simulink model "six_plus_six_AcmsteeringV09_main_2lfrf"  (R2014a)
settings: Solver=FixedStepDiscrete  StartTime=0.0  StopTime=10.0  FixedStep=0.0005  RelTol=1e-3
InitFcn:
  | Veh_Par_wxt
undefined symbols (not defined in the file or in its folder): acc_spdctl, ag_thr, B, bra_em, bra_pre_gz2, bra_pre_gz34, bra_pre_yd, brakepre_dem_data, brakeTrq_dem_data, bratrq_max, ecucoder_acal, eff_tran, ESP_switch, G, guzhang_lf, guzhang_lm, guzhang_lr, guzhang_rf, guzhang_rm, guzhang_rr, kd1, kd2, ki1, ki2, kp1, kp2, L, myFIS, premax, Radius, RC_switch, s_opt_yi, s_opt_zhuan, s_opt_zhuan_add, s_opt_zhuan_table, spd_map_mot, spd_spdctl, speed_thr_park, TCS_switch, tras_ratio, trq_map_mot, trqmax_yd, trqmax_zx, trqmaxneg, v_gain, v_table, v_thr_park, zhidong_bianmazhi, zhidong_down, zhidong_up, zhidong_youmen, zhuanxiang_bianmazhi, zhuanxiang_down, zhuanxiang_up, zhuanxiang_youmen
libraries: simulink x980, ec5744lib x59, fuzblock x2
(part 3 of 25)

== system six_plus_six_AcmsteeringV09_main_2lfrf/Data_input/MCU2_1 ==
  In1 : Inport
  In2 : Inport  Port=2
  Trigger : TriggerPort  TriggerType=function-call  PortDimensions=1
  MCU2 : Subsystem
  MCU2_MotorStallingFault : Outport
  MCU2_UdcDetectionFault : Outport  Port=2
  MCU2_TempSensorFault : Outport  Port=3
  MCU2_ActiveDischargingFault : Outport  Port=4
  MCU2_ldcSensorFault : Outport  Port=5
  MCU2_luSensorFault : Outport  Port=6
  MCU2_lvSensorFault : Outport  Port=7
  MCU2_FaultLevel : Outport  Port=8
  MCU2_Controllerload : Outport  Port=9
  MCU2_CanCommunicationFault : Outport  Port=10
  MCU2_MemoryFault : Outport  Port=11
  MCU2_DownratingFault : Outport  Port=12
  MCU2_IGBTFault : Outport  Port=13
  MCU2_MotorOverTemp : Outport  Port=14
  MCU2_ControllerOverTemp : Outport  Port=15
  MCU2_MotorOverSpeed : Outport  Port=16
  MCU2_RotaryInverterFault : Outport  Port=17
  MCU2_UnderVoltage : Outport  Port=18
  MCU2_OverVoltage : Outport  Port=19
  MCU2_MotorOverLoad : Outport  Port=20
  wires:
  MCU2/1(MCU2_MotorStallingFault_Out) -> MCU2_MotorStallingFault/1
  MCU2/7(MCU2_IvSensorFault_Out) -> MCU2_lvSensorFault/1
  MCU2/4(MCU2_ActieDischargingFault_Out) -> MCU2_ActiveDischargingFault/1
  MCU2/12(MCU2_DownratingFault_Out) -> MCU2_DownratingFault/1
  MCU2/13(MCU2_IGBTFault_Out) -> MCU2_IGBTFault/1
  MCU2/3(MCU2_TempSensorFault_Out) -> MCU2_TempSensorFault/1
  MCU2/10(MCU2_CanCommunicationFault_Out) -> MCU2_CanCommunicationFault/1
  MCU2/11(MCU2_MemoryFault_Out) -> MCU2_MemoryFault/1
  MCU2/14(MCU2_MotorOverTemp_Out) -> MCU2_MotorOverTemp/1
  MCU2/2(MCU2_UdcDetectionFault_Out) -> MCU2_UdcDetectionFault/1
  MCU2/5(MCU2_IdcSensorFault_Out) -> MCU2_ldcSensorFault/1
  In2/1 -> MCU2/1(input)
  In1/1 -> MCU2/Enable
  MCU2/6(MCU2_IuSensorFault_Out) -> MCU2_luSensorFault/1
  MCU2/8(MCU2_FaultLevel_Out) -> MCU2_FaultLevel/1
  MCU2/9(MCU2_ControllerOverload_Out) -> MCU2_Controllerload/1
  MCU2/20(MCU2_MotorOverLoad_Out) -> MCU2_MotorOverLoad/1
  MCU2/18(MCU2_UnderVoltage_Out) -> MCU2_UnderVoltage/1
  MCU2/19(MCU2_OverVoltage_Out) -> MCU2_OverVoltage/1
  MCU2/15(MCU2_ControllerOverTemp_Out) -> MCU2_ControllerOverTemp/1
  MCU2/16(MCU2_MotorOverSpeed_Out) -> MCU2_MotorOverSpeed/1
  MCU2/17(MCU2_RotaryInverterFault_Out) -> MCU2_RotaryInverterFault/1

== matlab function six_plus_six_AcmsteeringV09_main_2lfrf/MainControl/mode_control/backward/backward/Drive/驱动防滑控制TCS/直行TCS/直行/MATLAB Function7 ==
  data: trq_dem_lf input; trq_dem_lm input; trq_dem_lr input; trq_dem_rf input; trq_dem_rm input; trq_dem_rr input; bra_pre_l input; bra_pre_r input; brake_dem input; flag_lf input; flag_lm input; flag_lr input; trq_out_lf output; trq_out_lm output; flag_rf input; flag_rm input; flag_rr input; trq_out_lr output; trq_out_rf output; trq_out_rm output; trq_out_rr output; trq_pid_lf input; trq_pid_lm input; trq_pid_lr input; trq_pid_rf input; trq_pid_rm input; trq_pid_rr input; brapre_out_l output; brapre_out_r output; mode output
function [trq_out_lf,trq_out_lm,trq_out_lr,trq_out_rf,trq_out_rm,trq_out_rr,brapre_out_l,brapre_out_r,mode] = fcn(trq_dem_lf,trq_dem_lm,trq_dem_lr,trq_dem_rf,trq_dem_rm,trq_dem_rr,bra_pre_l,bra_pre_r,brake_dem,flag_lf,flag_lm,flag_lr,flag_rf,flag_rm,flag_rr,trq_pid_lf,trq_pid_lm,trq_pid_lr,trq_pid_rf,trq_pid_rm,trq_pid_rr)
%#codegen pid模块在外面做，里面进行十六种情况的判断，先看一下效果，不能再修改。
if flag_lf==0 && flag_lm==0 && flag_lr==0 && flag_rf==0 && flag_rm==0 && flag_rr==0 % 0电机滑转===============================================0电机滑转
    trq_out_lf=single(trq_dem_lf);
    trq_out_lm=single(trq_dem_lm);
    trq_out_lr=single(trq_dem_lr);
    trq_out_rf=single(trq_dem_rf);
    trq_out_rm=single(trq_dem_rm);
    trq_out_rr=single(trq_dem_rr);
    brapre_out_l=single(bra_pre_l+brake_dem);
    brapre_out_r=single(bra_pre_r+brake_dem);
    mode=int8(1);
    
    
    
    
    
    
    
    
    
elseif flag_lf==1 && flag_lm==0 && flag_lr==0 && flag_rf==0 && flag_rm==0 && flag_rr==0 %左前轮滑转===================================================1电机滑转
    trq_out_lf=single(trq_pid_lf);
    trq_out_lm=single(trq_dem_lm+(trq_dem_lf-trq_out_lf)/2);
    trq_out_lr=single(trq_dem_lr+(trq_dem_lf-trq_out_lf)/2);
    trq_out_rf=single(trq_dem_rf);
    trq_out_rm=single(trq_dem_rm);
    trq_out_rr=single(trq_dem_rr);
    brapre_out_l=single(bra_pre_l+brake_dem);
    brapre_out_r=single(bra_pre_r+brake_dem);
    mode=int8(2);
elseif flag_lf==0 && flag_lm==1 && flag_lr==0 && flag_rf==0 && flag_rm==0 && flag_rr==0 %左中轮滑转
    trq_out_lm=single(trq_pid_lm);
    trq_out_lf=single(trq_dem_lf+(trq_dem_lm-trq_out_lm)/2);
    trq_out_lr=single(trq_dem_lr+(trq_dem_lm-trq_out_lm)/2);
    trq_out_rf=single(trq_dem_rf);
    trq_out_rm=single(trq_dem_rm);
    trq_out_rr=single(trq_dem_rr);
    brapre_out_l=single(bra_pre_l+brake_dem);
    brapre_out_r=single(bra_pre_r+brake_dem);
    mode=int8(3);
elseif flag_lf==0 && flag_lm==0 && flag_lr==1 && flag_rf==0 && flag_rm==0 && flag_rr==0 %左后轮滑转
    trq_out_lr=single(trq_pid_lr);
    trq_out_lf=single(trq_dem_lf+(trq_dem_lr-trq_out_lr)/2);
    trq_out_lm=single(trq_dem_lm+(trq_dem_lr-trq_out_lr)/2);
    trq_out_rf=single(trq_dem_rf);
    trq_out_rm=single(trq_dem_rm);
    trq_out_rr=single(trq_dem_rr);
    brapre_out_l=single(bra_pre_l+brake_dem);
    brapre_out_r=single(bra_pre_r+brake_dem);
    mode=int8(4);
    
elseif flag_lf==0 && flag_lm==0 && flag_lr==0 && flag_rf==1 && flag_rm==0 && flag_rr==0 %右前轮滑转
    trq_out_rf=single(trq_pid_rf);
    trq_out_rm=single(trq_dem_rm+(trq_dem_rf-trq_out_rf)/2);
    trq_out_rr=single(trq_dem_rr+(trq_dem_rf-trq_out_rf)/2);
    trq_out_lf=single(trq_dem_lf);
    trq_out_lm=single(trq_dem_lm);
    trq_out_lr=single(trq_dem_lr);
    brapre_out_l=single(bra_pre_l+brake_dem);
    brapre_out_r=single(bra_pre_r+brake_dem);
    mode=int8(5);
elseif flag_lf==0 && flag_lm==0 && flag_lr==0 && flag_rf==0 && flag_rm==1 && flag_rr==0 %右中轮滑转
    trq_out_rm=single(trq_pid_rm);
    trq_out_rf=single(trq_dem_rf+(trq_dem_rm-trq_out_rm)/2);
    trq_out_rr=single(trq_dem_rr+(trq_dem_rm-trq_out_rm)/2);
    trq_out_lf=single(trq_dem_lf);
    trq_out_lm=single(trq_dem_lm);
    trq_out_lr=single(trq_dem_lr);
    brapre_out_l=single(bra_pre_l+brake_dem);
    brapre_out_r=single(bra_pre_r+brake_dem);
    mode=int8(6);
elseif flag_lf==0 && flag_lm==0 && flag_lr==0 && flag_rf==0 && flag_rm==0 && flag_rr==1 %右后轮滑转
    trq_out_rr=single(trq_pid_rr);
    trq_out_rf=single(trq_dem_rf+(trq_dem_rr-trq_out_rr)/2);
    trq_out_rm=single(trq_dem_rm+(trq_dem_rr-trq_out_rr)/2);
    trq_out_lf=single(trq_dem_lf);
    trq_out_lm=single(trq_dem_lm);
    trq_out_lr=single(trq_dem_lr);
    brapre_out_l=single(bra_pre_l+brake_dem);
    brapre_out_r=single(bra_pre_r+brake_dem);
    mode=int8(7);
    
    
    
    
    
    
    
    
    
    
elseif flag_lf==1 && flag_lm==1 && flag_lr==0 && flag_rf==0 && flag_rm==0 && flag_rr==0 %左前-左中 轮滑转===================================================2电机滑转    左侧
    trq_out_lf=single(trq_pid_lf);
    trq_out_lm=single(trq_pid_lm);
    trq_out_lr=single(trq_dem_lr+(trq_dem_lf-trq_out_lf)+(trq_dem_lm-trq_out_lm));
    trq_out_rf=single(trq_dem_rf);
    trq_out_rm=single(trq_dem_rm);
    trq_out_rr=single(trq_dem_rr);
    brapre_out_l=single(bra_pre_l+brake_dem);
    brapre_out_r=single(bra_pre_r+brake_dem);
    mode=int8(8);
elseif flag_lf==1 && flag_lm==0 && flag_lr==1 && flag_rf==0 && flag_rm==0 && flag_rr==0 %左前-左后 轮滑转
    trq_out_lf=single(trq_pid_lf);
    trq_out_lr=single(trq_pid_lr);
    trq_out_lm=single(trq_dem_lm+(trq_dem_lf-trq_out_lf)+(trq_dem_lr-trq_out_lr));
    trq_out_rf=single(trq_dem_rf);
    trq_out_rm=single(trq_dem_rm);
    trq_out_rr=single(trq_dem_rr);
    brapre_out_l=single(bra_pre_l+brake_dem);
    brapre_out_r=single(bra_pre_r+brake_dem);
    mode=int8(9);
elseif flag_lf==0 && flag_lm==1 && flag_lr==1 && flag_rf==0 && flag_rm==0 && flag_rr==0 %左中-左后 轮滑转
    trq_out_lm=single(trq_pid_lm);
    trq_out_lr=single(trq_pid_lr);
    trq_out_lf=single(trq_dem_lf+(trq_dem_lm-trq_out_lm)+(trq_dem_lr-trq_out_lr));
    trq_out_rf=single(trq_dem_rf);
    trq_out_rm=single(trq_dem_rm);
    trq_out_rr=single(trq_dem_rr);
    brapre_out_l=single(bra_pre_l+brake_dem);
    brapre_out_r=single(bra_pre_r+brake_dem);
    mode=int8(10);
    
elseif flag_lf==0 && flag_lm==0 && flag_lr==0 && flag_rf==1 && flag_rm==1 && flag_rr==0 %右前-右中 轮滑转                        右侧
    trq_out_rf=single(trq_pid_rf);
    trq_out_rm=single(trq_pid_rm);
    trq_out_rr=single(trq_dem_rr+(trq_dem_rf-trq_out_rf)+(trq_dem_rm-trq_out_rm));
    trq_out_lf=single(trq_dem_lf);
    trq_out_lm=single(trq_dem_lm);
    trq_out_lr=single(trq_dem_lr);
    brapre_out_l=single(bra_pre_l+brake_dem);
    brapre_out_r=single(bra_pre_r+brake_dem);
    mode=int8(11);
elseif flag_lf==0 && flag_lm==0 && flag_lr==0 && flag_rf==1 && flag_rm==0 && flag_rr==1 %右前-右后 轮滑转
    trq_out_rf=single(trq_pid_rf);
    trq_out_rr=single(trq_pid_rr);
    trq_out_rm=single(trq_dem_rm+(trq_dem_rf-trq_out_rf)+(trq_dem_rr-trq_out_rr));
    trq_out_lf=single(trq_dem_lf);
    trq_out_lm=single(trq_dem_lm);
    trq_out_lr=single(trq_dem_lr);
    brapre_out_l=single(bra_pre_l+brake_dem);
    brapre_out_r=single(bra_pre_r+brake_dem);
    mode=int8(12);
elseif flag_lf==0 && flag_lm==0 && flag_lr==0 && flag_rf==0 && flag_rm==1 && flag_rr==1 %右中-右后 轮滑转
    trq_out_rm=single(trq_pid_rm);
    trq_out_rr=single(trq_pid_rr);
    trq_out_rf=single(trq_dem_rf+(trq_dem_rm-trq_out_rm)+(trq_dem_rr-trq_out_rr));
    trq_out_lf=single(trq_dem_lf);
    trq_out_lm=single(trq_dem_lm);
    trq_out_lr=single(trq_dem_lr);
    brapre_out_l=single(bra_pre_l+brake_dem);
    brapre_out_r=single(bra_pre_r+brake_dem);
    mode=int8(13);
    
elseif flag_lf==1 && flag_lm==0 && flag_lr==0 && flag_rf==1 && flag_rm==0 && flag_rr==0 %左前-右前 轮滑转                 对侧
    trq_out_lf=single(trq_pid_lf);
    trq_out_lm=single(trq_dem_lm+(trq_dem_lf-trq_out_lf)/2);
    trq_out_lr=single(trq_dem_lr+(trq_dem_lf-trq_out_lf)/2);
    trq_out_rf=single(trq_pid_rf);
    trq_out_rm=single(trq_dem_rm+(trq_dem_rf-trq_out_rf)/2);
    trq_out_rr=single(trq_dem_rr+(trq_dem_rf-trq_out_rf)/2);
    brapre_out_l=single(bra_pre_l+brake_dem);
    brapre_out_r=single(bra_pre_r+brake_dem);
    mode=int8(14);
elseif flag_lf==1 && flag_lm==0 && flag_lr==0 && flag_rf==0 && flag_rm==1 && flag_rr==0 %左前-右中 轮滑转
    trq_out_lf=single(trq_pid_lf);
    trq_out_lm=single(trq_dem_lm+(trq_dem_lf-trq_out_lf)/2);
    trq_out_lr=single(trq_dem_lr+(trq_dem_lf-trq_out_lf)/2);
    trq_out_rm=single(trq_pid_rm);
    trq_out_rf=single(trq_dem_rf+(trq_dem_rm-trq_out_rm)/2);
    trq_out_rr=single(trq_dem_rr+(trq_dem_rm-trq_out_rm)/2);
    brapre_out_l=single(bra_pre_l+brake_dem);
    brapre_out_r=single(bra_pre_r+brake_dem);
    mode=int8(15);
elseif flag_lf==1 && flag_lm==0 && flag_lr==0 && flag_rf==0 && flag_rm==0 && flag_rr==1 %左前-右后 轮滑转
    trq_out_lf=single(trq_pid_lf);
    trq_out_lm=single(trq_dem_lm+(trq_dem_lf-trq_out_lf)/2);
    trq_out_lr=single(trq_dem_lr+(trq_dem_lf-trq_out_lf)/2);
    trq_out_rr=single(trq_pid_rr);
    trq_out_rf=single(trq_dem_rf+(trq_dem_rr-trq_out_rr)/2);
    trq_out_rm=single(trq_dem_rm+(trq_dem_rr-trq_out_rr)/2);
    brapre_out_l=single(bra_pre_l+brake_dem);
    brapre_out_r=single(bra_pre_r+brake_dem);
    mode=int8(16);
    
elseif flag_lf==0 && flag_lm==1 && flag_lr==0 && flag_rf==1 && flag_rm==0 && flag_rr==0 %左中-右前 轮滑转                 对侧
    trq_out_lm=single(trq_pid_lm);
    trq_out_lf=single(trq_dem_lf+(trq_dem_lm-trq_out_lm)/2);
    trq_out_lr=single(trq_dem_lr+(trq_dem_lm-trq_out_lm)/2);
    trq_out_rf=single(trq_pid_rf);
    trq_out_rm=single(trq_dem_rm+(trq_dem_rf-trq_out_rf)/2);
    trq_out_rr=single(trq_dem_rr+(trq_dem_rf-trq_out_rf)/2);
    brapre_out_l=single(bra_pre_l+brake_dem);
    brapre_out_r=single(bra_pre_r+brake_dem);
    mode=int8(17);
elseif flag_lf==0 && flag_lm==1 && flag_lr==0 && flag_rf==0 && flag_rm==1 && flag_rr==0 %左中-右中 轮滑转
    trq_out_lm=single(trq_pid_lm);
    trq_out_lf=single(trq_dem_lf+(trq_dem_lm-trq_out_lm)/2);
    trq_out_lr=single(trq_dem_lr+(trq_dem_lm-trq_out_lm)/2);
    trq_out_rm=single(trq_pid_rm);
    trq_out_rf=single(trq_dem_rf+(trq_dem_rm-trq_out_rm)/2);
    trq_out_rr=single(trq_dem_rr+(trq_dem_rm-trq_out_rm)/2);
    brapre_out_l=single(bra_pre_l+brake_dem);
    brapre_out_r=single(bra_pre_r+brake_dem);
    mode=int8(18);
elseif flag_lf==0 && flag_lm==1 && flag_lr==0 && flag_rf==0 && flag_rm==0 && flag_rr==1 %左中-右后 轮滑转
    trq_out_lm=single(trq_pid_lm);
    trq_out_lf=single(trq_dem_lf+(trq_dem_lm-trq_out_lm)/2);
    trq_out_lr=single(trq_dem_lr+(trq_dem_lm-trq_out_lm)/2);
    trq_out_rr=single(trq_pid_rr);
    trq_out_rf=single(trq_dem_rf+(trq_dem_rr-trq_out_rr)/2);
    trq_out_rm=single(trq_dem_rm+(trq_dem_rr-trq_out_rr)/2);
    brapre_out_l=single(bra_pre_l+brake_dem);
    brapre_out_r=single(bra_pre_r+brake_dem);
    mode=int8(19);
elseif flag_lf==0 && flag_lm==0 && flag_lr==1 && flag_rf==1 && flag_rm==0 && flag_rr==0 %左后-右前 轮滑转                 对侧
    trq_out_lr=single(trq_pid_lr);
    trq_out_lf=single(trq_dem_lf+(trq_dem_lr-trq_out_lr)/2);
    trq_out_lm=single(trq_dem_lm+(trq_dem_lr-trq_out_lr)/2);
    trq_out_rf=single(trq_pid_rf);
    trq_out_rm=single(trq_dem_rm+(trq_dem_rf-trq_out_rf)/2);
    trq_out_rr=single(trq_dem_rr+(trq_dem_rf-trq_out_rf)/2);
    brapre_out_l=single(bra_pre_l+brake_dem);
    brapre_out_r=single(bra_pre_r+brake_dem);
    mode=int8(20);
elseif flag_lf==0 && flag_lm==0 && flag_lr==1 && flag_rf==0 && flag_rm==1 && flag_rr==0 %左后-右中 轮滑转
    trq_out_lr=single(trq_pid_lr);
    trq_out_lf=single(trq_dem_lf+(trq_dem_lr-trq_out_lr)/2);
    trq_out_lm=single(trq_dem_lm+(trq_dem_lr-trq_out_lr)/2);
    trq_out_rm=single(trq_pid_rm);
    trq_out_rf=single(trq_dem_rf+(trq_dem_rm-trq_out_rm)/2);
    trq_out_rr=single(trq_dem_rr+(trq_dem_rm-trq_out_rm)/2);
    brapre_out_l=single(bra_pre_l+brake_dem);
    brapre_out_r=single(bra_pre_r+brake_dem);
    mode=int8(21);
elseif flag_lf==0 && flag_lm==0 && flag_lr==1 && flag_rf==0 && flag_rm==0 && flag_rr==1 %左后-右后 轮滑转
    trq_out_lr=single(trq_pid_lr);
    trq_out_lf=single(trq_dem_lf+(trq_dem_lr-trq_out_lr)/2);
    trq_out_lm=single(trq_dem_lm+(trq_dem_lr-trq_out_lr)/2);
    trq_out_rr=single(trq_pid_rr);
    trq_out_rf=single(trq_dem_rf+(trq_dem_rr-trq_out_rr)/2);
    trq_out_rm=single(trq_dem_rm+(trq_dem_rr-trq_out_rr)/2);
    brapre_out_l=single(bra_pre_l+brake_dem);
    brapre_out_r=single(bra_pre_r+brake_dem);
    mode=int8(22);
    
    
    
    
    
    
    
    
    
    
    
    
    
    
    
    
    
    
    
    
    
    
elseif flag_lf==1 && flag_lm==1 && flag_lr==1 && flag_rf==0 && flag_rm==0 && flag_rr==0 %左前-左中-左后 轮滑转===================================================3电机滑转    左侧
    trq_out_lf=single(trq_pid_lf);
    trq_out_lm=single(trq_pid_lm);
    trq_out_lr=single(trq_pid_lr);
    trq_out_rf=single(trq_dem_rf-((trq_dem_lf-trq_out_lf)+(trq_dem_lm-trq_out_lm)+(trq_dem_lr-trq_out_lr))/3);
    trq_out_rm=single(trq_dem_rm-((trq_dem_lf-trq_out_lf)+(trq_dem_lm-trq_out_lm)+(trq_dem_lr-trq_out_lr))/3);
    trq_out_rr=single(trq_dem_rr-((trq_dem_lf-trq_out_lf)+(trq_dem_lm-trq_out_lm)+(trq_dem_lr-trq_out_lr))/3);
    brapre_out_l=single(bra_pre_l+brake_dem);
    brapre_out_r=single(bra_pre_r+brake_dem);
    mode=int8(23);
elseif flag_lf==0 && flag_lm==0 && flag_lr==0 && flag_rf==1 && flag_rm==1 && flag_rr==1 %右前-右中-右后 轮滑转                      右侧
    trq_out_rf=single(trq_pid_rf);
    trq_out_rm=single(trq_pid_rm);
    trq_out_rr=single(trq_pid_rr);
    trq_out_lf=single(trq_dem_lf-((trq_dem_rf-trq_out_rf)+(trq_dem_rm-trq_out_rm)+(trq_dem_rr-trq_out_rr))/3);
    trq_out_lm=single(trq_dem_lm-((trq_dem_rf-trq_out_rf)+(trq_dem_rm-trq_out_rm)+(trq_dem_rr-trq_out_rr))/3);
    trq_out_lr=single(trq_dem_lr-((trq_dem_rf-trq_out_rf)+(trq_dem_rm-trq_out_rm)+(trq_dem_rr-trq_out_rr))/3);
    brapre_out_l=single(bra_pre_l+brake_dem);
    brapre_out_r=single(bra_pre_r+brake_dem);
    mode=int8(24);
    
elseif flag_lf==1 && flag_lm==1 && flag_lr==0 && flag_rf==1 && flag_rm==0 && flag_rr==0 %左前-左中-右前 轮滑转
    trq_out_lf=single(trq_pid_lf);
    trq_out_lm=single(trq_pid_lm);
    trq_out_lr=single(trq_dem_lr+(trq_dem_lf-trq_out_lf)+(trq_dem_lm-trq_out_lm));
    trq_out_rf=single(trq_pid_rf);
    trq_out_rm=single(trq_dem_rm+(trq_dem_rf-trq_out_rf)/2);
    trq_out_rr=single(trq_dem_rr+(trq_dem_rf-trq_out_rf)/2);
    brapre_out_l=single(bra_pre_l+brake_dem);
    brapre_out_r=single(bra_pre_r+brake_dem);
    mode=int8(25);
elseif flag_lf==1 && flag_lm==1 && flag_lr==0 && flag_rf==0 && flag_rm==1 && flag_rr==0 %左前-左中-右中 轮滑转
    trq_out_lf=single(trq_pid_lf);
    trq_out_lm=single(trq_pid_lm);
    trq_out_lr=single(trq_dem_lr+(trq_dem_lf-trq_out_lf)+(trq_dem_lm-trq_out_lm));
    trq_out_rm=single(trq_pid_rm);
    trq_out_rf=single(trq_dem_rf+(trq_dem_rm-trq_out_rm)/2);
    trq_out_rr=single(trq_dem_rr+(trq_dem_rm-trq_out_rm)/2);
    brapre_out_l=single(bra_pre_l+brake_dem);
    brapre_out_r=single(bra_pre_r+brake_dem);
    mode=int8(26);
elseif flag_lf==1 && flag_lm==1 && flag_lr==0 && flag_rf==0 && flag_rm==0 && flag_rr==1 %左前-左中-右后 轮滑转
    trq_out_lf=single(trq_pid_lf);
    trq_out_lm=single(trq_pid_lm);
    trq_out_lr=single(trq_dem_lr+(trq_dem_lf-trq_out_lf)+(trq_dem_lm-trq_out_lm));
    trq_out_rr=single(trq_pid_rr);
    trq_out_rf=single(trq_dem_rf+(trq_dem_rr-trq_out_rr)/2);
    trq_out_rm=single(trq_dem_rm+(trq_dem_rr-trq_out_rr)/2);
    brapre_out_l=single(bra_pre_l+brake_dem);
    brapre_out_r=single(bra_pre_r+brake_dem);
    mode=int8(27);
    
elseif flag_lf==1 && flag_lm==0 && flag_lr==1 && flag_rf==1 && flag_rm==0 && flag_rr==0 %左前-左后-右前 轮滑转
    trq_out_lf=single(trq_pid_lf);
    trq_out_lr=single(trq_pid_lr);
    trq_out_lm=single(trq_dem_lm+(trq_dem_lf-trq_out_lf)+(trq_dem_lr-trq_out_lr));
    trq_out_rf=single(trq_pid_rf);
    trq_out_rm=single(trq_dem_rm+(trq_dem_rf-trq_out_rf)/2);
    trq_out_rr=single(trq_dem_rr+(trq_dem_rf-trq_out_rf)/2);
    brapre_out_l=single(bra_pre_l+brake_dem);
    brapre_out_r=single(bra_pre_r+brake_dem);
    mode=int8(28);
elseif flag_lf==1 && flag_lm==0 && flag_lr==1 && flag_rf==0 && flag_rm==1 && flag_rr==0 %左前-左后-右中 轮滑转
    trq_out_lf=single(trq_pid_lf);
    trq_out_lr=single(trq_pid_lr);
    trq_out_lm=single(trq_dem_lm+(trq_dem_lf-trq_out_lf)+(trq_dem_lr-trq_out_lr));
    trq_out_rm=single(trq_pid_rm);
    trq_out_rf=single(trq_dem_rf+(trq_dem_rm-trq_out_rm)/2);
    trq_out_rr=single(trq_dem_rr+(trq_dem_rm-trq_out_rm)/2);
    brapre_out_l=single(bra_pre_l+brake_dem);
    brapre_out_r=single(bra_pre_r+brake_dem);
    mode=int8(29);
elseif flag_lf==1 && flag_lm==0 && flag_lr==1 && flag_rf==0 && flag_rm==0 && flag_rr==1 %左前-左后-右后 轮滑转
    trq_out_lf=single(trq_pid_lf);
    trq_out_lr=single(trq_pid_lr);
    trq_out_lm=single(trq_dem_lm+(trq_dem_lf-trq_out_lf)+(trq_dem_lr-trq_out_lr));
    trq_out_rr=single(trq_pid_rr);
    trq_out_rf=single(trq_dem_rf+(trq_dem_rr-trq_out_rr)/2);
    trq_out_rm=single(trq_dem_rm+(trq_dem_rr-trq_out_rr)/2);
    brapre_out_l=single(bra_pre_l+brake_dem);
    brapre_out_r=single(bra_pre_r+brake_dem);
    mode=int8(30);
    
elseif flag_lf==0 && flag_lm==1 && flag_lr==1 && flag_rf==1 && flag_rm==0 && flag_rr==0 %左中-左后-右前 轮滑转
    trq_out_lm=single(trq_pid_lm);
    trq_out_lr=single(trq_pid_lr);
    trq_out_lf=single(trq_dem_lf+(trq_dem_lm-trq_out_lm)+(trq_dem_lr-trq_out_lr));
    trq_out_rf=single(trq_pid_rf);
    trq_out_rm=single(trq_dem_rm+(trq_dem_rf-trq_out_rf)/2);
    trq_out_rr=single(trq_dem_rr+(trq_dem_rf-trq_out_rf)/2);
    brapre_out_l=single(bra_pre_l+brake_dem);
    brapre_out_r=single(bra_pre_r+brake_dem);
    mode=int8(31);
elseif flag_lf==0 && flag_lm==1 && flag_lr==1 && flag_rf==0 && flag_rm==1 && flag_rr==0 %左中-左后-右中 轮滑转
    trq_out_lm=single(trq_pid_lm);
    trq_out_lr=single(trq_pid_lr);
    trq_out_lf=single(trq_dem_lf+(trq_dem_lm-trq_out_lm)+(trq_dem_lr-trq_out_lr));
    trq_out_rm=single(trq_pid_rm);
    trq_out_rf=single(trq_dem_rf+(trq_dem_rm-trq_out_rm)/2);
    trq_out_rr=single(trq_dem_rr+(trq_dem_rm-trq_out_rm)/2);
    brapre_out_l=single(bra_pre_l+brake_dem);
    brapre_out_r=single(bra_pre_r+brake_dem);
    mode=int8(32);
elseif flag_lf==0 && flag_lm==1 && flag_lr==1 && flag_rf==0 && flag_rm==0 && flag_rr==1 %左中-左后-右后 轮滑转
    trq_out_lm=single(trq_pid_lm);
    trq_out_lr=single(trq_pid_lr);
    trq_out_lf=single(trq_dem_lf+(trq_dem_lm-trq_out_lm)+(trq_dem_lr-trq_out_lr));
    trq_out_rr=single(trq_pid_rr);
    trq_out_rf=single(trq_dem_rf+(trq_dem_rr-trq_out_rr)/2);
    trq_out_rm=single(trq_dem_rm+(trq_dem_rr-trq_out_rr)/2);
    brapre_out_l=single(bra_pre_l+brake_dem);
    brapre_out_r=single(bra_pre_r+brake_dem);
    mode=int8(33);
    
elseif flag_lf==1 && flag_lm==0 && flag_lr==0 && flag_rf==1 && flag_rm==1 && flag_rr==0 %右前-右中-左前 轮滑转
    trq_out_rf=single(trq_pid_rf);
    trq_out_rm=single(trq_pid_rm);
    trq_out_rr=single(trq_dem_rr+(trq_dem_rf-trq_out_rf)+(trq_dem_rm-trq_out_rm));
    trq_out_lf=single(trq_pid_lf);
    trq_out_lm=single(trq_dem_lm+(trq_dem_lf-trq_out_lf)/2);
    trq_out_lr=single(trq_dem_lr+(trq_dem_lf-trq_out_lf)/2);
    brapre_out_l=single(bra_pre_l+brake_dem);
    brapre_out_r=single(bra_pre_r+brake_dem);
    mode=int8(34);
elseif flag_lf==0 && flag_lm==1 && flag_lr==0 && flag_rf==1 && flag_rm==1 && flag_rr==0 %右前-右中-左中 轮滑转
    trq_out_rf=single(trq_pid_rf);
    trq_out_rm=single(trq_pid_rm);
    trq_out_rr=single(trq_dem_rr+(trq_dem_rf-trq_out_rf)+(trq_dem_rm-trq_out_rm));
    trq_out_lm=single(trq_pid_lm);
    trq_out_lf=single(trq_dem_lf+(trq_dem_lm-trq_out_lm)/2);
    trq_out_lr=single(trq_dem_lr+(trq_dem_lm-trq_out_lm)/2);
    brapre_out_l=single(bra_pre_l+brake_dem);
    brapre_out_r=single(bra_pre_r+brake_dem);
    mode=int8(35);
elseif flag_lf==0 && flag_lm==0 && flag_lr==1 && flag_rf==1 && flag_rm==1 && flag_rr==0 %右前-右中-左后 轮滑转
    trq_out_rf=single(trq_pid_rf);
    trq_out_rm=single(trq_pid_rm);
    trq_out_rr=single(trq_dem_rr+(trq_dem_rf-trq_out_rf)+(trq_dem_rm-trq_out_rm));
    trq_out_lr=single(trq_pid_lr);
    trq_out_lf=single(trq_dem_lf+(trq_dem_lr-trq_out_lr)/2);
    trq_out_lm=single(trq_dem_lm+(trq_dem_lr-trq_out_lr)/2);
    brapre_out_l=single(bra_pre_l+brake_dem);
    brapre_out_r=single(bra_pre_r+brake_dem);
    mode=int8(36);
    
elseif flag_lf==1 && flag_lm==0 && flag_lr==0 && flag_rf==1 && flag_rm==0 && flag_rr==1 %右前-右后-左前 轮滑转
    trq_out_rf=single(trq_pid_rf);
    trq_out_rr=single(trq_pid_rr);
    trq_out_rm=single(trq_dem_rm+(trq_dem_rf-trq_out_rf)+(trq_dem_rr-trq_out_rr));
    trq_out_lf=single(trq_pid_lf);
    trq_out_lm=single(trq_dem_lm+(trq_dem_lf-trq_out_lf)/2);
    trq_out_lr=single(trq_dem_lr+(trq_dem_lf-trq_out_lf)/2);
    brapre_out_l=single(bra_pre_l+brake_dem);
    brapre_out_r=single(bra_pre_r+brake_dem);
    mode=int8(37);
elseif flag_lf==0 && flag_lm==1 && flag_lr==0 && flag_rf==1 && flag_rm==0 && flag_rr==1 %右前-右后-左中 轮滑转
    trq_out_rf=single(trq_pid_rf);
    trq_out_rr=single(trq_pid_rr);
    trq_out_rm=single(trq_dem_rm+(trq_dem_rf-trq_out_rf)+(trq_dem_rr-trq_out_rr));
    trq_out_lm=single(trq_pid_lm);
    trq_out_lf=single(trq_dem_lf+(trq_dem_lm-trq_out_lm)/2);
    trq_out_lr=single(trq_dem_lr+(trq_dem_lm-trq_out_lm)/2);
    brapre_out_l=single(bra_pre_l+brake_dem);
    brapre_out_r=single(bra_pre_r+brake_dem);
    mode=int8(38);
elseif flag_lf==0 && flag_lm==0 && flag_lr==1 && flag_rf==1 && flag_rm==0 && flag_rr==1 %右前-右后-左后 轮滑转
    trq_out_rf=single(trq_pid_rf);
    trq_out_rr=single(trq_pid_rr);
    trq_out_rm=single(trq_dem_rm+(trq_dem_rf-trq_out_rf)+(trq_dem_rr-trq_out_rr));
    trq_out_lr=single(trq_pid_lr);
    trq_out_lf=single(trq_dem_lf+(trq_dem_lr-trq_out_lr)/2);
    trq_out_lm=single(trq_dem_lm+(trq_dem_lr-trq_out_lr)/2);
    brapre_out_l=single(bra_pre_l+brake_dem);
    brapre_out_r=single(bra_pre_r+brake_dem);
    mode=int8(39);
    
elseif flag_lf==1 && flag_lm==0 && flag_lr==0 && flag_rf==0 && flag_rm==1 && flag_rr==1 %右中-右后-左前 轮滑转
    trq_out_rm=single(trq_pid_rm);
    trq_out_rr=single(trq_pid_rr);
    trq_out_rf=single(trq_dem_rf+(trq_dem_rm-trq_out_rm)+(trq_dem_rr-trq_out_rr));
    trq_out_lf=single(trq_pid_lf);
    trq_out_lm=single(trq_dem_lm+(trq_dem_lf-trq_out_lf)/2);
    trq_out_lr=single(trq_dem_lr+(trq_dem_lf-trq_out_lf)/2);
    brapre_out_l=single(bra_pre_l+brake_dem);
    brapre_out_r=single(bra_pre_r+brake_dem);
    mode=int8(40);
elseif flag_lf==0 && flag_lm==1 && flag_lr==0 && flag_rf==0 && flag_rm==1 && flag_rr==1 %右中-右后-左中 轮滑转
    trq_out_rm=single(trq_pid_rm);
    trq_out_rr=single(trq_pid_rr);
    trq_out_rf=single(trq_dem_rf+(trq_dem_rm-trq_out_rm)+(trq_dem_rr-trq_out_rr));
    trq_out_lm=single(trq_pid_lm);
    trq_out_lf=single(trq_dem_lf+(trq_dem_lm-trq_out_lm)/2);
    trq_out_lr=single(trq_dem_lr+(trq_dem_lm-trq_out_lm)/2);
    brapre_out_l=single(bra_pre_l+brake_dem);
    brapre_out_r=single(bra_pre_r+brake_dem);
    mode=int8(41);
elseif flag_lf==0 && flag_lm==0 && flag_lr==1 && flag_rf==0 && flag_rm==1 && flag_rr==1 %右中-右后-左后 轮滑转
    trq_out_rm=single(trq_pid_rm);
    trq_out_rr=single(trq_pid_rr);
    trq_out_rf=single(trq_dem_rf+(trq_dem_rm-trq_out_rm)+(trq_dem_rr-trq_out_rr));
    trq_out_lr=single(trq_pid_lr);
    trq_out_lf=single(trq_dem_lf+(trq_dem_lr-trq_out_lr)/2);
    trq_out_lm=single(trq_dem_lm+(trq_dem_lr-trq_out_lr)/2);
    brapre_out_l=single(bra_pre_l+brake_dem);
    brapre_out_r=single(bra_pre_r+brake_dem);
    mode=int8(42);
    
    
    
    
    
    
    
    
    
    
    
    
    
    
    
    
    
    
    
    
    
elseif flag_lf==1 && flag_lm==1 && flag_lr==1 && flag_rf==1 && flag_rm==0 && flag_rr==0 %左前-左中-左后 右前 轮滑转===================================================4电机滑转
    trq_out_lf=single(trq_pid_lf);
    trq_out_lm=single(trq_pid_lm);
    trq_out_lr=single(trq_pid_lr);
    trq_out_rf=single(trq_pid_rf);
    trq_out_rm=single(trq_dem_rm-((trq_dem_lf-trq_out_lf)+(trq_dem_lm-trq_out_lm)+(trq_dem_lr-trq_out_lr)-(trq_dem_rf-trq_out_rf))/2);
    trq_out_rr=single(trq_dem_rr-((trq_dem_lf-trq_out_lf)+(trq_dem_lm-trq_out_lm)+(trq_dem_lr-trq_out_lr)-(trq_dem_rf-trq_out_rf))/2);
    brapre_out_l=single(bra_pre_l+brake_dem);
    brapre_out_r=single(bra_pre_r+brake_dem);
    mode=int8(43);
elseif flag_lf==1 && flag_lm==1 && flag_lr==1 && flag_rf==0 && flag_rm==1 && flag_rr==0 %左前-左中-左后 右中 轮滑转
    trq_out_lf=single(trq_pid_lf);
    trq_out_lm=single(trq_pid_lm);
    trq_out_lr=single(trq_pid_lr);
    trq_out_rm=single(trq_pid_rm);
    trq_out_rf=single(trq_dem_rf-((trq_dem_lf-trq_out_lf)+(trq_dem_lm-trq_out_lm)+(trq_dem_lr-trq_out_lr)-(trq_dem_rm-trq_out_rm))/2);
    trq_out_rr=single(trq_dem_rr-((trq_dem_lf-trq_out_lf)+(trq_dem_lm-trq_out_lm)+(trq_dem_lr-trq_out_lr)-(trq_dem_rm-trq_out_rm))/2);
    brapre_out_l=single(bra_pre_l+brake_dem);
    brapre_out_r=single(bra_pre_r+brake_dem);
    mode=int8(44);
elseif flag_lf==1 && flag_lm==1 && flag_lr==1 && flag_rf==0 && flag_rm==0 && flag_rr==1 %左前-左中-左后 右后 轮滑转
    trq_out_lf=single(trq_pid_lf);
    trq_out_lm=single(trq_pid_lm);
    trq_out_lr=single(trq_pid_lr);
    trq_out_rr=single(trq_pid_rr);
    trq_out_rf=single(trq_dem_rf-((trq_dem_lf-trq_out_lf)+(trq_dem_lm-trq_out_lm)+(trq_dem_lr-trq_out_lr)-(trq_dem_rr-trq_out_rr))/2);
    trq_out_rm=single(trq_dem_rm-((trq_dem_lf-trq_out_lf)+(trq_dem_lm-trq_out_lm)+(trq_dem_lr-trq_out_lr)-(trq_dem_rr-trq_out_rr))/2);
    brapre_out_l=single(bra_pre_l+brake_dem);
    brapre_out_r=single(bra_pre_r+brake_dem);
    mode=int8(45);
    
elseif flag_lf==1 && flag_lm==0 && flag_lr==0 && flag_rf==1 && flag_rm==1 && flag_rr==1 %右前-右中-右后 左前 轮滑转
    trq_out_rf=single(trq_pid_rf);
    trq_out_rm=single(trq_pid_rm);
    trq_out_rr=single(trq_pid_rr);
    trq_out_lf=single(trq_pid_lf);
    trq_out_lm=single(trq_dem_lm-((trq_dem_rf-trq_out_rf)+(trq_dem_rm-trq_out_rm)+(trq_dem_rr-trq_out_rr)-(trq_dem_lf-trq_out_lf))/2);
    trq_out_lr=single(trq_dem_lr-((trq_dem_rf-trq_out_rf)+(trq_dem_rm-trq_out_rm)+(trq_dem_rr-trq_out_rr)-(trq_dem_lf-trq_out_lf))/2);
    brapre_out_l=single(bra_pre_l+brake_dem);
    brapre_out_r=single(bra_pre_r+brake_dem);
    mode=int8(46);
elseif flag_lf==0 && flag_lm==1 && flag_lr==0 && flag_rf==1 && flag_rm==1 && flag_rr==1 %右前-右中-右后 左中 轮滑转
    trq_out_rf=single(trq_pid_rf);
    trq_out_rm=single(trq_pid_rm);
    trq_out_rr=single(trq_pid_rr);
    trq_out_lm=single(trq_pid_lm);
    trq_out_lf=single(trq_dem_lf-((trq_dem_rf-trq_out_rf)+(trq_dem_rm-trq_out_rm)+(trq_dem_rr-trq_out_rr)-(trq_dem_lm-trq_out_lm))/2);
    trq_out_lr=single(trq_dem_lr-((trq_dem_rf-trq_out_rf)+(trq_dem_rm-trq_out_rm)+(trq_dem_rr-trq_out_rr)-(trq_dem_lm-trq_out_lm))/2);
    brapre_out_l=single(bra_pre_l+brake_dem);
    brapre_out_r=single(bra_pre_r+brake_dem);
    mode=int8(47);
elseif flag_lf==0 && flag_lm==0 && flag_lr==1 && flag_rf==1 && flag_rm==1 && flag_rr==1 %右前-右中-右后 左后 轮滑转
    trq_out_rf=single(trq_pid_rf);
    trq_out_rm=single(trq_pid_rm);
    trq_out_rr=single(trq_pid_rr);
    trq_out_lr=single(trq_pid_lr);
    trq_out_lf=single(trq_dem_lf-((trq_dem_rf-trq_out_rf)+(trq_dem_rm-trq_out_rm)+(trq_dem_rr-trq_out_rr)-(trq_dem_lr-trq_out_lr))/2);
    trq_out_lm=single(trq_dem_lm-((trq_dem_rf-trq_out_rf)+(trq_dem_rm-trq_out_rm)+(trq_dem_rr-trq_out_rr)-(trq_dem_lr-trq_out_lr))/2);
    brapre_out_l=single(bra_pre_l+brake_dem);
    brapre_out_r=single(bra_pre_r+brake_dem);
    mode=int8(48);
    
elseif flag_lf==1 && flag_lm==1 && flag_lr==0 && flag_rf==1 && flag_rm==1 && flag_rr==0 %左前-左中 右前-右中 轮滑转
    trq_out_lf=single(trq_pid_lf);
    trq_out_lm=single(trq_pid_lm);
    trq_out_lr=single(trq_dem_lr+(trq_dem_lf-trq_out_lf)+(trq_dem_lm-trq_out_lm));
    trq_out_rf=single(trq_pid_rf);
    trq_out_rm=single(trq_pid_rm);
    trq_out_rr=single(trq_dem_rr+(trq_dem_rf-trq_out_rf)+(trq_dem_rm-trq_out_rm));
    brapre_out_l=single(bra_pre_l+brake_dem);
    brapre_out_r=single(bra_pre_r+brake_dem);
    mode=int8(49);
elseif flag_lf==1 && flag_lm==1 && flag_lr==0 && flag_rf==1 && flag_rm==0 && flag_rr==1 %左前-左中 右前-右后 轮滑转
    trq_out_lf=single(trq_pid_lf);
    trq_out_lm=single(trq_pid_lm);
    trq_out_lr=single(trq_dem_lr+(trq_dem_lf-trq_out_lf)+(trq_dem_lm-trq_out_lm));
    trq_out_rf=single(trq_pid_rf);
    trq_out_rr=single(trq_pid_rr);
    trq_out_rm=single(trq_dem_rm+(trq_dem_rf-trq_out_rf)+(trq_dem_rr-trq_out_rr));
    brapre_out_l=single(bra_pre_l+brake_dem);
    brapre_out_r=single(bra_pre_r+brake_dem);
    mode=int8(50);
elseif flag_lf==1 && flag_lm==1 && flag_lr==0 && flag_rf==0 && flag_rm==1 && flag_rr==1 %左前-左中 右中-右后 轮滑转
    trq_out_lf=single(trq_pid_lf);
    trq_out_lm=single(trq_pid_lm);
    trq_out_lr=single(trq_dem_lr+(trq_dem_lf-trq_out_lf)+(trq_dem_lm-trq_out_lm));
    trq_out_rm=single(trq_pid_rm);
    trq_out_rr=single(trq_pid_rr);
    trq_out_rf=single(trq_dem_rf+(trq_dem_rm-trq_out_rm)+(trq_dem_rr-trq_out_rr));
    brapre_out_l=single(bra_pre_l+brake_dem);
    brapre_out_r=single(bra_pre_r+brake_dem);
    mode=int8(51);
    
elseif flag_lf==1 && flag_lm==0 && flag_lr==1 && flag_rf==1 && flag_rm==1 && flag_rr==0 %左前-左后 右前-右中 轮滑转
    trq_out_lf=single(trq_pid_lf);
    trq_out_lr=single(trq_pid_lr);
    trq_out_lm=single(trq_dem_lm+(trq_dem_lf-trq_out_lf)+(trq_dem_lr-trq_out_lr));
    trq_out_rf=single(trq_pid_rf);
    trq_out_rm=single(trq_pid_rm);
    trq_out_rr=single(trq_dem_rr+(trq_dem_rf-trq_out_rf)+(trq_dem_rm-trq_out_rm));
    brapre_out_l=single(bra_pre_l+brake_dem);
    brapre_out_r=single(bra_pre_r+brake_dem);
    mode=int8(52);
elseif flag_lf==1 && flag_lm==0 && flag_lr==1 && flag_rf==1 && flag_rm==0 && flag_rr==1 %左前-左后 右前-右后 轮滑转
    trq_out_lf=single(trq_pid_lf);
    trq_out_lr=single(trq_pid_lr);
    trq_out_lm=single(trq_dem_lm+(trq_dem_lf-trq_out_lf)+(trq_dem_lr-trq_out_lr));
    trq_out_rf=single(trq_pid_rf);
    trq_out_rr=single(trq_pid_rr);
    trq_out_rm=single(trq_dem_rm+(trq_dem_rf-trq_out_rf)+(trq_dem_rr-trq_out_rr));
    brapre_out_l=single(bra_pre_l+brake_dem);
    brapre_out_r=single(bra_pre_r+brake_dem);
    mode=int8(53);
elseif flag_lf==1 && flag_lm==0 && flag_lr==1 && flag_rf==0 && flag_rm==1 && flag_rr==1 %左前-左后 右中-右后 轮滑转
    trq_out_lf=single(trq_pid_lf);
    trq_out_lr=single(trq_pid_lr);
    trq_out_lm=single(trq_dem_lm+(trq_dem_lf-trq_out_lf)+(trq_dem_lr-trq_out_lr));
    trq_out_rm=single(trq_pid_rm);
    trq_out_rr=single(trq_pid_rr);
    trq_out_rf=single(trq_dem_rf+(trq_dem_rm-trq_out_rm)+(trq_dem_rr-trq_out_rr));
    brapre_out_l=single(bra_pre_l+brake_dem);
    brapre_out_r=single(bra_pre_r+brake_dem);
    mode=int8(54);
    
elseif flag_lf==0 && flag_lm==1 && flag_lr==1 && flag_rf==1 && flag_rm==1 && flag_rr==0 %左中-左后 右前-右中 轮滑转
    trq_out_lm=single(trq_pid_lm);
    trq_out_lr=single(trq_pid_lr);
    trq_out_lf=single(trq_dem_lf+(trq_dem_lm-trq_out_lm)+(trq_dem_lr-trq_out_lr));
    trq_out_rf=single(trq_pid_rf);
    trq_out_rm=single(trq_pid_rm);
    trq_out_rr=single(trq_dem_rr+(trq_dem_rf-trq_out_rf)+(trq_dem_rm-trq_out_rm));
    brapre_out_l=single(bra_pre_l+brake_dem);
    brapre_out_r=single(bra_pre_r+brake_dem);
    mode=int8(55);
elseif flag_lf==0 && flag_lm==1 && flag_lr==1 && flag_rf==1 && flag_rm==0 && flag_rr==1 %左中-左后 右前-右后 轮滑转
    trq_out_lm=single(trq_pid_lm);
    trq_out_lr=single(trq_pid_lr);
    trq_out_lf=single(trq_dem_lf+(trq_dem_lm-trq_out_lm)+(trq_dem_lr-trq_out_lr));
    trq_out_rf=single(trq_pid_rf);
    trq_out_rr=single(trq_pid_rr);
    trq_out_rm=single(trq_dem_rm+(trq_dem_rf-trq_out_rf)+(trq_dem_rr-trq_out_rr));
    brapre_out_l=single(bra_pre_l+brake_dem);
    brapre_out_r=single(bra_pre_r+brake_dem);
    mode=int8(56);
elseif flag_lf==0 && flag_lm==1 && flag_lr==1 && flag_rf==0 && flag_rm==1 && flag_rr==1 %左中-左后 右中-右后 轮滑转
    trq_out_lm=single(trq_pid_lm);
    trq_out_lr=single(trq_pid_lr);
    trq_out_lf=single(trq_dem_lf+(trq_dem_lm-trq_out_lm)+(trq_dem_lr-trq_out_lr));
    trq_out_rm=single(trq_pid_rm);
    trq_out_rr=single(trq_pid_rr);
    trq_out_rf=single(trq_dem_rf+(trq_dem_rm-trq_out_rm)+(trq_dem_rr-trq_out_rr));
    brapre_out_l=single(bra_pre_l+brake_dem);
    brapre_out_r=single(bra_pre_r+brake_dem);
    mode=int8(57);
    
    
    
    
    
    
    
    
    
    
    
    
    
    
    
    
    
elseif flag_lf==1 && flag_lm==1 && flag_lr==1 && flag_rf==1 && flag_rm==1 && flag_rr==0 %右后轮不划转===================================================5电机滑转
    trq_out_lf=single(trq_pid_lf);
    trq_out_lm=single(trq_pid_lm);
    trq_out_lr=single(trq_pid_lr);
    trq_out_rf=single(trq_pid_rf);
    trq_out_rm=single(trq_pid_rm);
    trq_out_rr=single(trq_dem_rr-((trq_dem_lf-trq_out_lf)+(trq_dem_lm-trq_out_lm)+(trq_dem_lr-trq_out_lr)-(trq_dem_rf-trq_out_rf)-(trq_dem_rm-trq_out_rm)));
    brapre_out_l=single(bra_pre_l+brake_dem);
    brapre_out_r=single(bra_pre_r+brake_dem);
    mode=int8(58);
elseif flag_lf==1 && flag_lm==1 && flag_lr==1 && flag_rf==1 && flag_rm==0 && flag_rr==1 %右中轮不划转
    trq_out_lf=single(trq_pid_lf);
    trq_out_lm=single(trq_pid_lm);
    trq_out_lr=single(trq_pid_lr);
    trq_out_rf=single(trq_pid_rf);
    trq_out_rr=single(trq_pid_rr);
    trq_out_rm=single(trq_dem_rm-((trq_dem_lf-trq_out_lf)+(trq_dem_lm-trq_out_lm)+(trq_dem_lr-trq_out_lr)-(trq_dem_rf-trq_out_rf)-(trq_dem_rr-trq_out_rr)));
    brapre_out_l=single(bra_pre_l+brake_dem);
    brapre_out_r=single(bra_pre_r+brake_dem);
    mode=int8(59);
elseif flag_lf==1 && flag_lm==1 && flag_lr==1 && flag_rf==0 && flag_rm==1 && flag_rr==1 %右前轮不划转
    trq_out_lf=single(trq_pid_lf);
    trq_out_lm=single(trq_pid_lm);
    trq_out_lr=single(trq_pid_lr);
    trq_out_rm=single(trq_pid_rm);
    trq_out_rr=single(trq_pid_rr);
    trq_out_rf=single(trq_dem_rf-((trq_dem_lf-trq_out_lf)+(trq_dem_lm-trq_out_lm)+(trq_dem_lr-trq_out_lr)-(trq_dem_rm-trq_out_rm)-(trq_dem_rr-trq_out_rr)));
    brapre_out_l=single(bra_pre_l+brake_dem);
    brapre_out_r=single(bra_pre_r+brake_dem);
    mode=int8(60);
elseif flag_lf==1 && flag_lm==1 && flag_lr==0 && flag_rf==1 && flag_rm==1 && flag_rr==1 %左后轮不划转===================================================5电机滑转
    trq_out_rf=single(trq_pid_rf);
    trq_out_rm=single(trq_pid_rm);
    trq_out_rr=single(trq_pid_rr);
    trq_out_lf=single(trq_pid_lf);
    trq_out_lm=single(trq_pid_lm);
    trq_out_lr=single(trq_dem_lr-((trq_dem_rf-trq_out_rf)+(trq_dem_rm-trq_out_rm)+(trq_dem_rr-trq_out_rr)-(trq_dem_lf-trq_out_lf)-(trq_dem_lm-trq_out_lm)));
    brapre_out_l=single(bra_pre_l+brake_dem);
    brapre_out_r=single(bra_pre_r+brake_dem);
    mode=int8(61);
elseif flag_lf==1 && flag_lm==0 && flag_lr==1 && flag_rf==1 && flag_rm==1 && flag_rr==1 %左中轮不划转
    trq_out_rf=single(trq_pid_rf);
    trq_out_rm=single(trq_pid_rm);
    trq_out_rr=single(trq_pid_rr);
    trq_out_lf=single(trq_pid_lf);
    trq_out_lr=single(trq_pid_lr);
    trq_out_lm=single(trq_dem_lm-((trq_dem_rf-trq_out_rf)+(trq_dem_rm-trq_out_rm)+(trq_dem_rr-trq_out_rr)-(trq_dem_lf-trq_out_lf)-(trq_dem_lr-trq_out_lr)));
    brapre_out_l=single(bra_pre_l+brake_dem);
    brapre_out_r=single(bra_pre_r+brake_dem);
    mode=int8(62);
elseif flag_lf==0 && flag_lm==1 && flag_lr==1 && flag_rf==1 && flag_rm==1 && flag_rr==1 %左前轮不划转
    trq_out_rf=single(trq_pid_rf);
    trq_out_rm=single(trq_pid_rm);
    trq_out_rr=single(trq_pid_rr);
    trq_out_lm=single(trq_pid_lm);
    trq_out_lr=single(trq_pid_lr);
    trq_out_lf=single(trq_dem_lf-((trq_dem_rf-trq_out_rf)+(trq_dem_rm-trq_out_rm)+(trq_dem_rr-trq_out_rr)-(trq_dem_lm-trq_out_lm)-(trq_dem_lr-trq_out_lr)));
    brapre_out_l=single(bra_pre_l+brake_dem);
    brapre_out_r=single(bra_pre_r+brake_dem);
    mode=int8(63);
    
    
    
    
    
    
    
    
    
    
    
    
    
else
    %     flag_lf==1 && flag_lm==1 && flag_lr==1 && flag_rf==1 && flag_rm==1 && flag_rr==1 %===================================================6电机滑转
    trq_out_lf=single(trq_pid_lf);
    trq_out_lm=single(trq_pid_lm);
    trq_out_lr=single(trq_pid_lr);
    trq_out_rf=single(trq_pid_rf);
    trq_out_rm=single(trq_pid_rm);
    trq_out_rr=single(trq_pid_rr);
    trqcha=(trq_dem_lf-trq_out_lf)+(trq_dem_lm-trq_out_lm)+(trq_dem_lr-trq_out_lr)-(trq_dem_rf-trq_out_rf)-(trq_dem_rm-trq_out_rm)-(trq_dem_rr-trq_out_rr);
    if trqcha>=0
        trq_out_rf=trq_pid_rf-trqcha/3;
        trq_out_rm=trq_pid_rm-trqcha/3;
        trq_out_rr=trq_pid_rr-trqcha/3;
    else
        trq_out_lf=trq_pid_lf+trqcha/3;
        trq_out_lm=trq_pid_lm+trqcha/3;
        trq_out_lr=trq_pid_lr+trqcha/3;
    end
    brapre_out_l=single(bra_pre_l+brake_dem);
    brapre_out_r=single(bra_pre_r+brake_dem);
    mode=int8(64);
end



trq_out_lf=single(trq_out_lf);
trq_out_lm=single(trq_out_lm);
trq_out_lr=single(trq_out_lr);
trq_out_rf=single(trq_out_rf);
trq_out_rm=single(trq_out_rm);
trq_out_rr=single(trq_out_rr);
brapre_out_l=single(brapre_out_l);
brapre_out_r=single(brapre_out_r);
end

== system six_plus_six_AcmsteeringV09_main_2lfrf/Data_input/MCU2_2 ==
  In1 : Inport
  In2 : Inport  Port=2
  Trigger : TriggerPort  TriggerType=function-call  PortDimensions=1
  MCU2 : Subsystem
  MCU2_MotorStallingFault : Outport
  MCU2_UdcDetectionFault : Outport  Port=2
  MCU2_TempSensorFault : Outport  Port=3
  MCU2_ActiveDischargingFault : Outport  Port=4
  MCU2_ldcSensorFault : Outport  Port=5
  MCU2_luSensorFault : Outport  Port=6
  MCU2_lvSensorFault : Outport  Port=7
  MCU2_FaultLevel : Outport  Port=8
  MCU2_Controllerload : Outport  Port=9
  MCU2_CanCommunicationFault : Outport  Port=10
  MCU2_MemoryFault : Outport  Port=11
  MCU2_DownratingFault : Outport  Port=12
  MCU2_IGBTFault : Outport  Port=13
  MCU2_MotorOverTemp : Outport  Port=14
  MCU2_ControllerOverTemp : Outport  Port=15
  MCU2_MotorOverSpeed : Outport  Port=16
  MCU2_RotaryInverterFault : Outport  Port=17
  MCU2_UnderVoltage : Outport  Port=18
  MCU2_OverVoltage : Outport  Port=19
  MCU2_MotorOverLoad : Outport  Port=20
  wires:
  MCU2/1(MCU2_MotorStallingFault_Out) -> MCU2_MotorStallingFault/1
  MCU2/7(MCU2_IvSensorFault_Out) -> MCU2_lvSensorFault/1
  MCU2/4(MCU2_ActieDischargingFault_Out) -> MCU2_ActiveDischargingFault/1
  MCU2/12(MCU2_DownratingFault_Out) -> MCU2_DownratingFault/1
  MCU2/13(MCU2_IGBTFault_Out) -> MCU2_IGBTFault/1
  MCU2/3(MCU2_TempSensorFault_Out) -> MCU2_TempSensorFault/1
  MCU2/10(MCU2_CanCommunicationFault_Out) -> MCU2_CanCommunicationFault/1
  MCU2/11(MCU2_MemoryFault_Out) -> MCU2_MemoryFault/1
  MCU2/14(MCU2_MotorOverTemp_Out) -> MCU2_MotorOverTemp/1
  MCU2/2(MCU2_UdcDetectionFault_Out) -> MCU2_UdcDetectionFault/1
  MCU2/5(MCU2_IdcSensorFault_Out) -> MCU2_ldcSensorFault/1
  In2/1 -> MCU2/1(input)
  In1/1 -> MCU2/Enable
  MCU2/6(MCU2_IuSensorFault_Out) -> MCU2_luSensorFault/1
  MCU2/8(MCU2_FaultLevel_Out) -> MCU2_FaultLevel/1
  MCU2/9(MCU2_ControllerOverload_Out) -> MCU2_Controllerload/1
  MCU2/20(MCU2_MotorOverLoad_Out) -> MCU2_MotorOverLoad/1
  MCU2/18(MCU2_UnderVoltage_Out) -> MCU2_UnderVoltage/1
  MCU2/19(MCU2_OverVoltage_Out) -> MCU2_OverVoltage/1
  MCU2/15(MCU2_ControllerOverTemp_Out) -> MCU2_ControllerOverTemp/1
  MCU2/16(MCU2_MotorOverSpeed_Out) -> MCU2_MotorOverSpeed/1
  MCU2/17(MCU2_RotaryInverterFault_Out) -> MCU2_RotaryInverterFault/1

== system six_plus_six_AcmsteeringV09_main_2lfrf/Data_input/MCU2_3 ==
  In1 : Inport
  In2 : Inport  Port=2
  Trigger : TriggerPort  TriggerType=function-call  PortDimensions=1
  MCU2 : Subsystem
  MCU2_MotorStallingFault : Outport
  MCU2_UdcDetectionFault : Outport  Port=2
  MCU2_TempSensorFault : Outport  Port=3
  MCU2_ActiveDischargingFault : Outport  Port=4
  MCU2_ldcSensorFault : Outport  Port=5
  MCU2_luSensorFault : Outport  Port=6
  MCU2_lvSensorFault : Outport  Port=7
  MCU2_FaultLevel : Outport  Port=8
  MCU2_Controllerload : Outport  Port=9
  MCU2_CanCommunicationFault : Outport  Port=10
  MCU2_MemoryFault : Outport  Port=11
  MCU2_DownratingFault : Outport  Port=12
  MCU2_IGBTFault : Outport  Port=13
  MCU2_MotorOverTemp : Outport  Port=14
  MCU2_ControllerOverTemp : Outport  Port=15
  MCU2_MotorOverSpeed : Outport  Port=16
  MCU2_RotaryInverterFault : Outport  Port=17
  MCU2_UnderVoltage : Outport  Port=18
  MCU2_OverVoltage : Outport  Port=19
  MCU2_MotorOverLoad : Outport  Port=20
  wires:
  MCU2/1(MCU2_MotorStallingFault_Out) -> MCU2_MotorStallingFault/1
  MCU2/7(MCU2_IvSensorFault_Out) -> MCU2_lvSensorFault/1
  MCU2/4(MCU2_ActieDischargingFault_Out) -> MCU2_ActiveDischargingFault/1
  MCU2/12(MCU2_DownratingFault_Out) -> MCU2_DownratingFault/1
  MCU2/13(MCU2_IGBTFault_Out) -> MCU2_IGBTFault/1
  MCU2/3(MCU2_TempSensorFault_Out) -> MCU2_TempSensorFault/1
  MCU2/10(MCU2_CanCommunicationFault_Out) -> MCU2_CanCommunicationFault/1
  MCU2/11(MCU2_MemoryFault_Out) -> MCU2_MemoryFault/1
  MCU2/14(MCU2_MotorOverTemp_Out) -> MCU2_MotorOverTemp/1
  MCU2/2(MCU2_UdcDetectionFault_Out) -> MCU2_UdcDetectionFault/1
  MCU2/5(MCU2_IdcSensorFault_Out) -> MCU2_ldcSensorFault/1
  In2/1 -> MCU2/1(input)
  In1/1 -> MCU2/Enable
  MCU2/6(MCU2_IuSensorFault_Out) -> MCU2_luSensorFault/1
  MCU2/8(MCU2_FaultLevel_Out) -> MCU2_FaultLevel/1
  MCU2/9(MCU2_ControllerOverload_Out) -> MCU2_Controllerload/1
  MCU2/20(MCU2_MotorOverLoad_Out) -> MCU2_MotorOverLoad/1
  MCU2/18(MCU2_UnderVoltage_Out) -> MCU2_UnderVoltage/1
  MCU2/19(MCU2_OverVoltage_Out) -> MCU2_OverVoltage/1
  MCU2/15(MCU2_ControllerOverTemp_Out) -> MCU2_ControllerOverTemp/1
  MCU2/16(MCU2_MotorOverSpeed_Out) -> MCU2_MotorOverSpeed/1
  MCU2/17(MCU2_RotaryInverterFault_Out) -> MCU2_RotaryInverterFault/1

== system six_plus_six_AcmsteeringV09_main_2lfrf/Data_input/MCU2_4 ==
  In1 : Inport
  In2 : Inport  Port=2
  Trigger : TriggerPort  TriggerType=function-call  PortDimensions=1
  MCU2 : Subsystem
  MCU2_MotorStallingFault : Outport
  MCU2_UdcDetectionFault : Outport  Port=2
  MCU2_TempSensorFault : Outport  Port=3
  MCU2_ActiveDischargingFault : Outport  Port=4
  MCU2_ldcSensorFault : Outport  Port=5
  MCU2_luSensorFault : Outport  Port=6
  MCU2_lvSensorFault : Outport  Port=7
  MCU2_FaultLevel : Outport  Port=8
  MCU2_Controllerload : Outport  Port=9
  MCU2_CanCommunicationFault : Outport  Port=10
  MCU2_MemoryFault : Outport  Port=11
  MCU2_DownratingFault : Outport  Port=12
  MCU2_IGBTFault : Outport  Port=13
  MCU2_MotorOverTemp : Outport  Port=14
  MCU2_ControllerOverTemp : Outport  Port=15
  MCU2_MotorOverSpeed : Outport  Port=16
  MCU2_RotaryInverterFault : Outport  Port=17
  MCU2_UnderVoltage : Outport  Port=18
  MCU2_OverVoltage : Outport  Port=19
  MCU2_MotorOverLoad : Outport  Port=20
  wires:
  MCU2/1(MCU2_MotorStallingFault_Out) -> MCU2_MotorStallingFault/1
  MCU2/7(MCU2_IvSensorFault_Out) -> MCU2_lvSensorFault/1
  MCU2/4(MCU2_ActieDischargingFault_Out) -> MCU2_ActiveDischargingFault/1
  MCU2/12(MCU2_DownratingFault_Out) -> MCU2_DownratingFault/1
  MCU2/13(MCU2_IGBTFault_Out) -> MCU2_IGBTFault/1
  MCU2/3(MCU2_TempSensorFault_Out) -> MCU2_TempSensorFault/1
  MCU2/10(MCU2_CanCommunicationFault_Out) -> MCU2_CanCommunicationFault/1
  MCU2/11(MCU2_MemoryFault_Out) -> MCU2_MemoryFault/1
  MCU2/14(MCU2_MotorOverTemp_Out) -> MCU2_MotorOverTemp/1
  MCU2/2(MCU2_UdcDetectionFault_Out) -> MCU2_UdcDetectionFault/1
  MCU2/5(MCU2_IdcSensorFault_Out) -> MCU2_ldcSensorFault/1
  In2/1 -> MCU2/1(input)
  In1/1 -> MCU2/Enable
  MCU2/6(MCU2_IuSensorFault_Out) -> MCU2_luSensorFault/1
  MCU2/8(MCU2_FaultLevel_Out) -> MCU2_FaultLevel/1
  MCU2/9(MCU2_ControllerOverload_Out) -> MCU2_Controllerload/1
  MCU2/20(MCU2_MotorOverLoad_Out) -> MCU2_MotorOverLoad/1
  MCU2/18(MCU2_UnderVoltage_Out) -> MCU2_UnderVoltage/1
  MCU2/19(MCU2_OverVoltage_Out) -> MCU2_OverVoltage/1
  MCU2/15(MCU2_ControllerOverTemp_Out) -> MCU2_ControllerOverTemp/1
  MCU2/16(MCU2_MotorOverSpeed_Out) -> MCU2_MotorOverSpeed/1
  MCU2/17(MCU2_RotaryInverterFault_Out) -> MCU2_RotaryInverterFault/1

== system six_plus_six_AcmsteeringV09_main_2lfrf/Data_input/MCU2_5 ==
  In1 : Inport
  In2 : Inport  Port=2
  Trigger : TriggerPort  TriggerType=function-call  PortDimensions=1
  MCU2 : Subsystem
  MCU2_MotorStallingFault : Outport
  MCU2_UdcDetectionFault : Outport  Port=2
  MCU2_TempSensorFault : Outport  Port=3
  MCU2_ActiveDischargingFault : Outport  Port=4
  MCU2_ldcSensorFault : Outport  Port=5
  MCU2_luSensorFault : Outport  Port=6
  MCU2_lvSensorFault : Outport  Port=7
  MCU2_FaultLevel : Outport  Port=8
  MCU2_Controllerload : Outport  Port=9
  MCU2_CanCommunicationFault : Outport  Port=10
  MCU2_MemoryFault : Outport  Port=11
  MCU2_DownratingFault : Outport  Port=12
  MCU2_IGBTFault : Outport  Port=13
  MCU2_MotorOverTemp : Outport  Port=14
  MCU2_ControllerOverTemp : Outport  Port=15
  MCU2_MotorOverSpeed : Outport  Port=16
  MCU2_RotaryInverterFault : Outport  Port=17
  MCU2_UnderVoltage : Outport  Port=18
  MCU2_OverVoltage : Outport  Port=19
  MCU2_MotorOverLoad : Outport  Port=20
  wires:
  MCU2/1(MCU2_MotorStallingFault_Out) -> MCU2_MotorStallingFault/1
  MCU2/7(MCU2_IvSensorFault_Out) -> MCU2_lvSensorFault/1
  MCU2/4(MCU2_ActieDischargingFault_Out) -> MCU2_ActiveDischargingFault/1
  MCU2/12(MCU2_DownratingFault_Out) -> MCU2_DownratingFault/1
  MCU2/13(MCU2_IGBTFault_Out) -> MCU2_IGBTFault/1
  MCU2/3(MCU2_TempSensorFault_Out) -> MCU2_TempSensorFault/1
  MCU2/10(MCU2_CanCommunicationFault_Out) -> MCU2_CanCommunicationFault/1
  MCU2/11(MCU2_MemoryFault_Out) -> MCU2_MemoryFault/1
  MCU2/14(MCU2_MotorOverTemp_Out) -> MCU2_MotorOverTemp/1
  MCU2/2(MCU2_UdcDetectionFault_Out) -> MCU2_UdcDetectionFault/1
  MCU2/5(MCU2_IdcSensorFault_Out) -> MCU2_ldcSensorFault/1
  In2/1 -> MCU2/1(input)
  In1/1 -> MCU2/Enable
  MCU2/6(MCU2_IuSensorFault_Out) -> MCU2_luSensorFault/1
  MCU2/8(MCU2_FaultLevel_Out) -> MCU2_FaultLevel/1
  MCU2/9(MCU2_ControllerOverload_Out) -> MCU2_Controllerload/1
  MCU2/20(MCU2_MotorOverLoad_Out) -> MCU2_MotorOverLoad/1
  MCU2/18(MCU2_UnderVoltage_Out) -> MCU2_UnderVoltage/1
  MCU2/19(MCU2_OverVoltage_Out) -> MCU2_OverVoltage/1
  MCU2/15(MCU2_ControllerOverTemp_Out) -> MCU2_ControllerOverTemp/1
  MCU2/16(MCU2_MotorOverSpeed_Out) -> MCU2_MotorOverSpeed/1
  MCU2/17(MCU2_RotaryInverterFault_Out) -> MCU2_RotaryInverterFault/1

== system six_plus_six_AcmsteeringV09_main_2lfrf/Data_input/RemoteControl1 ==
  In1 : Inport
  In2 : Inport  Port=2
  Trigger : TriggerPort  TriggerType=function-call  PortDimensions=1
  Yaokong2 : Subsystem
  SH : Outport
  SE : Outport  Port=2
  SD : Outport  Port=3
  SA : Outport  Port=4
  LIFEspan : Outport  Port=5
  wires:
  Yaokong2/2(SE_Out) -> SE/1
  Yaokong2/3(SD_Out) -> SD/1
  Yaokong2/4(SA_Out) -> SA/1
  In2/1 -> Yaokong2/1(input)
  In1/1 -> Yaokong2/Enable
  Yaokong2/1(SH_Out) -> SH/1
  Yaokong2/5(LIFEspan_Out) -> LIFEspan/1
